simulink model "ControlPD"  (R2021a)
settings: Solver=ode4  StartTime=0.0  StopTime=20  FixedStep=0.01  RelTol=1e-3
settings Model: PauseTimes=10  Creator=benja  LastModifiedBy=benja

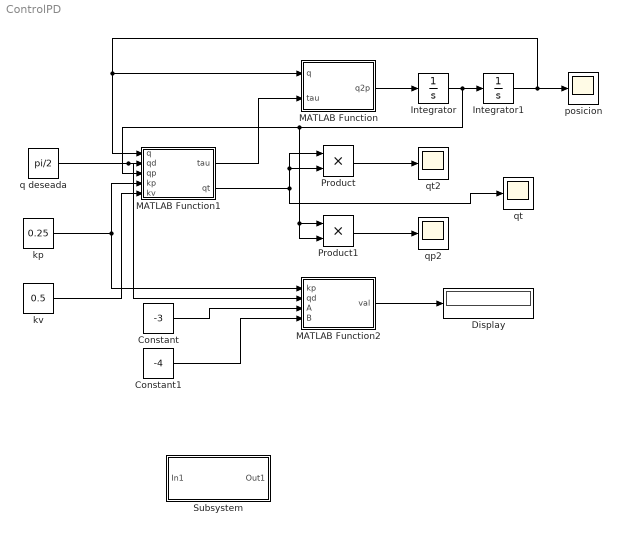
== system ControlPD ==
  Constant : Constant  Value=-3
  Constant1 : Constant  Value=-4
  Display : Display
  Integrator : Integrator
  Integrator1 : Integrator
  MATLAB Function : MATLAB Function  TreatAsAtomicUnit=on
  MATLAB Function1 : MATLAB Function  TreatAsAtomicUnit=on
  MATLAB Function2 : MATLAB Function  TreatAsAtomicUnit=on
  Product : Product
  Product1 : Product
  Subsystem : Subsystem
  kp : Constant  Value=0.25
  kv : Constant  Value=0.5
  posicion : Scope
  q deseada : Constant  Value=pi/2
  qp2 : Scope
  qt : Scope
  qt2 : Scope
  wires:
  MATLAB Function/1(q2p) -> Integrator/1
  Integrator/1 -> MATLAB Function1/3(qp), Product1/1, Product1/2, Integrator1/1
  Integrator1/1 -> posicion/1, MATLAB Function1/1(q), MATLAB Function/1(q)
  MATLAB Function1/1(tau) -> MATLAB Function/2(tau)
  kp/1 -> MATLAB Function2/1(kp), MATLAB Function1/4(kp)
  kv/1 -> MATLAB Function1/5(kv)
  MATLAB Function1/2(qt) -> qt/1, Product/1, Product/2
  Product/1 -> qt2/1
  Product1/1 -> qp2/1
  q deseada/1 -> MATLAB Function2/2(qd), MATLAB Function1/2(qd)
  Constant/1 -> MATLAB Function2/3(A)
  Constant1/1 -> MATLAB Function2/4(B)
  MATLAB Function2/1(val) -> Display/1

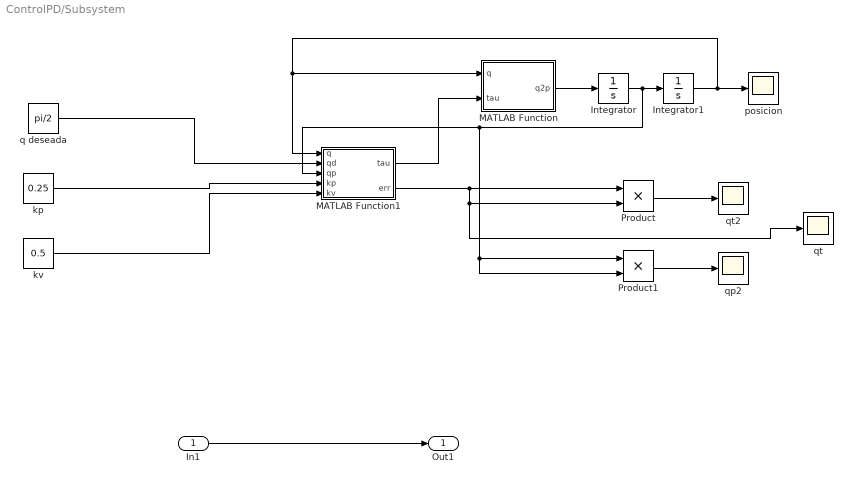
== system ControlPD/Subsystem ==
  In1 : Inport
  Integrator : Integrator
  Integrator1 : Integrator
  MATLAB Function : MATLAB Function  TreatAsAtomicUnit=on
  MATLAB Function1 : MATLAB Function  TreatAsAtomicUnit=on
  Product : Product
  Product1 : Product
  kp : Constant  Value=0.25
  kv : Constant  Value=0.5
  posicion : Scope
  q deseada : Constant  Value=pi/2
  qp2 : Scope
  qt : Scope
  qt2 : Scope
  Out1 : Outport
  wires:
  In1/1 -> Out1/1
  kp/1 -> MATLAB Function1/4(kp)
  Integrator1/1 -> posicion/1, MATLAB Function1/1(q), MATLAB Function/1(q)
  Product/1 -> qt2/1
  MATLAB Function1/2(err) -> Product/2, qt/1, Product/1
  MATLAB Function1/1(tau) -> MATLAB Function/2(tau)
  Product1/1 -> qp2/1
  q deseada/1 -> MATLAB Function1/2(qd)
  kv/1 -> MATLAB Function1/5(kv)
  MATLAB Function/1(q2p) -> Integrator/1
  Integrator/1 -> MATLAB Function1/3(qp), Product1/1, Product1/2, Integrator1/1

== matlab function ControlPD/MATLAB Function1 ==
  data: q input; tau output; qd input; qp input; kp input; kv input; qt output
function [tau,qt] = fcn(q,qd,qp,kp,kv)

qt = qd - q;
tau = kp*qt-kv*qp;

== matlab function ControlPD/MATLAB Function ==
  data: q input; q2p output; tau input
function q2p = fcn(q,tau)

m = 1;
g = 1;
l = 1;
q2p =inv(m*l)*(tau-m*g*l*sin(q));

== matlab function ControlPD/MATLAB Function2 ==
  data: kp input; val output; qd input; A input; B input
function val = fcn(kp,qd,A,B)
    coder.extrinsic('biseccionFunc');
    persistent val2
    persistent var
    val = 0
    if isempty(var)
        var = 1
        val2 = biseccionFunc(kp,qd,double(A),double(B));   	            
    end
    val = val2

== matlab function ControlPD/Subsystem/MATLAB Function ==
  data: q input; q2p output; tau input
function q2p = fcn(q,tau)

m = 1;
g = 1;
l = 1;
q2p =inv(m*l)*(tau-m*g*l*sin(q));

== matlab function ControlPD/Subsystem/MATLAB Function1 ==
  data: q input; tau output; qd input; qp input; kp input; kv input; err output
function [tau,err] = fcn(q,qd,qp,kp,kv)

err = qd - q;
tau = kp*err-kv*qp;
